simulink model "pod_3_level_V1_2"  (R2018a)
settings: Solver=VariableStepAuto  StartTime=0.0  StopTime=0.1  RelTol=1e-3
libraries: powerlib x24, simulink x6
settings Model: Creator=SuperITCom  LastModifiedBy=SuperITCom

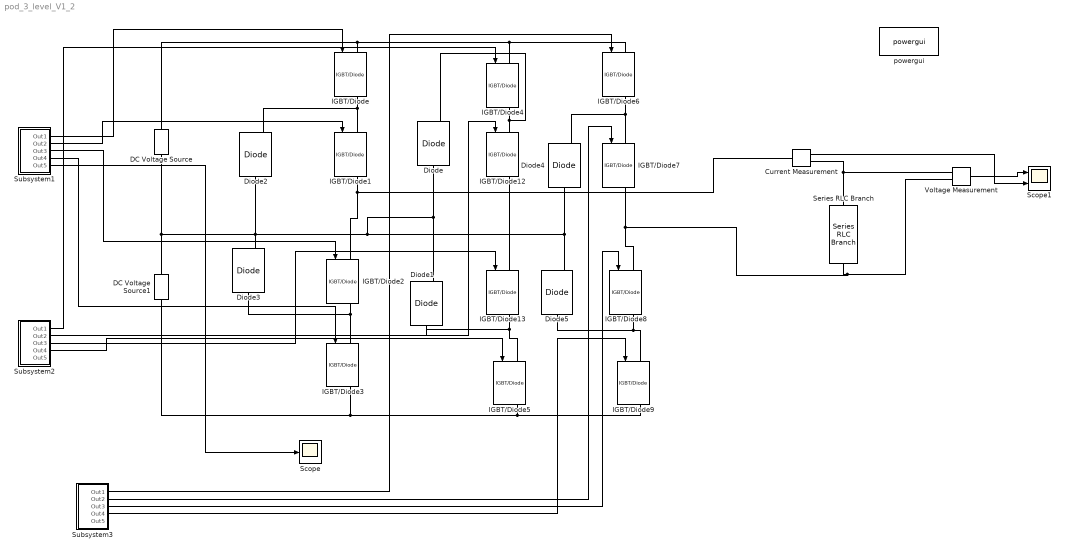
== system pod_3_level_V1_2 ==
  Current Measurement : powerlib/Measurements/Current Measurement  PhasorSimulation=off  OutputType=Complex  PSBequivalent=0
  DC Voltage Source : powerlib/Electrical Sources/DC Voltage Source  Amplitude=200  Measurements=None
  DC Voltage Source1 : powerlib/Electrical Sources/DC Voltage Source  Amplitude=200  Measurements=None
  Diode{,1..5} (6 alike) : powerlib/Power Electronics/Diode  Ron=0.001  Lon=0  Vf=0.8  IC=0  UseSnubber=0  Rs=500  Cs=250e-9  Measurements=on
  IGBT/Diode{,1..9,12..13} (12 alike) : powerlib/Power Electronics/IGBT//Diode  Ron=1e-3  Rs=1e5  Cs=inf  Measurements=on
  Scope : Scope
  Scope1 : Scope  NumInputPorts=2
  Series RLC Branch : powerlib/Elements/Series RLC Branch  LConnTagsString=__new0  RConnTagsString=__new0  BranchType=RL  Resistance=5  Inductance=5e-3  SetiL0=off  InitialCurrent=0  Capacitance=5e-3  Setx0=off  InitialVoltage=0  Measurements=None
  Subsystem1 : Subsystem
  Subsystem2 : Subsystem
  Subsystem3 : Subsystem
  Voltage Measurement : powerlib/Measurements/Voltage Measurement  PhasorSimulation=off  OutputType=Complex  PSBequivalent=0
  powergui : powerlib/powergui  Priority=1  SimulationMode=Discrete  SampleTime=50e-6  frequency=60  Iterations=50  frequencyindice=0  Pbase=100e6  ErrMax=1e-4  UnitsV=kV  UnitsW=MW  buscounter=0  FunctionMessages=off  echomessages=off  EnableUseOfTLC=off  CurrentSourceSwitches=off  DisableSnubberDevices=off  DisableRonSwitches=off  DisableVfSwitches=off  DisplayEquations=off  SolverType=Tustin/Backward Euler (TBE)  Interpol=off  ExternalGateDelay=off  methode=off  Ts=100  x0status=blocks  SPID=off  SwTol=0  HookPort=off  RestoreLinks=warning  ResistiveCurrentMeasurement=off  Frange=[0:2:500]  Ylog=off  Xlog=on  ShowGrid=off  save=off  variable=ZData  structure=linevoltpod3  ZoomFFT=on  StartTime=0.0  cycles=2  DisplayStyle=1  fundamental=50  FreqAxis=on  MaxFrequency=1000  frequencyindicesteady=1  RmsSteady=1  display=off
  wires:
  Current Measurement/1 -> Scope1/2
  Subsystem2/3(Out3) -> IGBT/Diode13/1
  Subsystem1/2(Out2) -> IGBT/Diode1/1
  Subsystem1/5(Out5) -> Scope/1
  Subsystem3/3(Out3) -> IGBT/Diode8/1
  Subsystem1/4(Out4) -> IGBT/Diode3/1
  Subsystem2/4(Out4) -> IGBT/Diode5/1
  Voltage Measurement/1 -> Scope1/1
  Subsystem1/1(Out1) -> IGBT/Diode/1
  Subsystem2/2(Out2) -> IGBT/Diode12/1
  Subsystem3/1(Out1) -> IGBT/Diode6/1
  Subsystem3/4(Out4) -> IGBT/Diode9/1
  Subsystem1/3(Out3) -> IGBT/Diode2/1
  Subsystem3/2(Out2) -> IGBT/Diode7/1
  Subsystem2/1(Out1) -> IGBT/Diode4/1
  connections:
  IGBT/Diode/LConn1 -- DC Voltage Source/RConn1 -- IGBT/Diode4/LConn1 -- IGBT/Diode6/LConn1
  Diode2/LConn1 -- Diode1/RConn1 -- Diode/LConn1 -- Diode4/LConn1 -- Diode5/RConn1 -- DC Voltage Source1/RConn1 -- DC Voltage Source/LConn1 -- Diode3/RConn1
  IGBT/Diode5/RConn1 -- IGBT/Diode3/RConn1 -- DC Voltage Source1/LConn1 -- IGBT/Diode9/RConn1
  IGBT/Diode12/LConn1 -- IGBT/Diode4/RConn1 -- Diode/RConn1
  IGBT/Diode2/LConn1 -- Current Measurement/LConn1 -- IGBT/Diode1/RConn1
  Series RLC Branch/LConn1 -- Current Measurement/RConn1 -- Voltage Measurement/LConn1
  IGBT/Diode2/RConn1 -- Diode3/LConn1 -- IGBT/Diode3/LConn1
  IGBT/Diode1/LConn1 -- IGBT/Diode/RConn1 -- Diode2/RConn1
  IGBT/Diode5/LConn1 -- IGBT/Diode13/RConn1 -- Diode1/LConn1
  Diode5/LConn1 -- IGBT/Diode9/LConn1 -- IGBT/Diode8/RConn1
  IGBT/Diode7/LConn1 -- IGBT/Diode6/RConn1 -- Diode4/RConn1
  IGBT/Diode12/RConn1 -- IGBT/Diode13/LConn1
  IGBT/Diode7/RConn1 -- Series RLC Branch/RConn1 -- Voltage Measurement/LConn2 -- IGBT/Diode8/LConn1

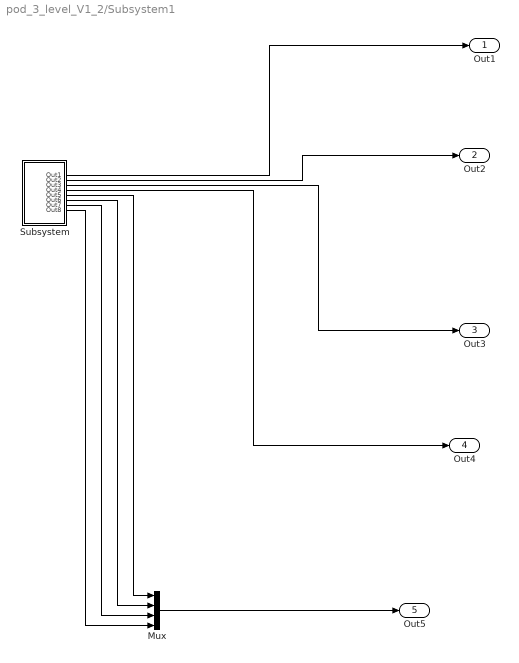
== system pod_3_level_V1_2/Subsystem1 ==
  Mux : Mux
  Subsystem : Subsystem
  Out1 : Outport
  Out2 : Outport  Port=2
  Out3 : Outport  Port=3
  Out4 : Outport  Port=4
  Out5 : Outport  Port=5
  wires:
  Subsystem/6(Out6) -> Mux/2
  Subsystem/5(Out5) -> Mux/1
  Subsystem/8(Out8) -> Mux/4
  Subsystem/7(Out7) -> Mux/3
  Subsystem/1(Out1) -> Out1/1
  Mux/1 -> Out5/1
  Subsystem/2(Out2) -> Out2/1
  Subsystem/4(Out4) -> Out4/1
  Subsystem/3(Out3) -> Out3/1

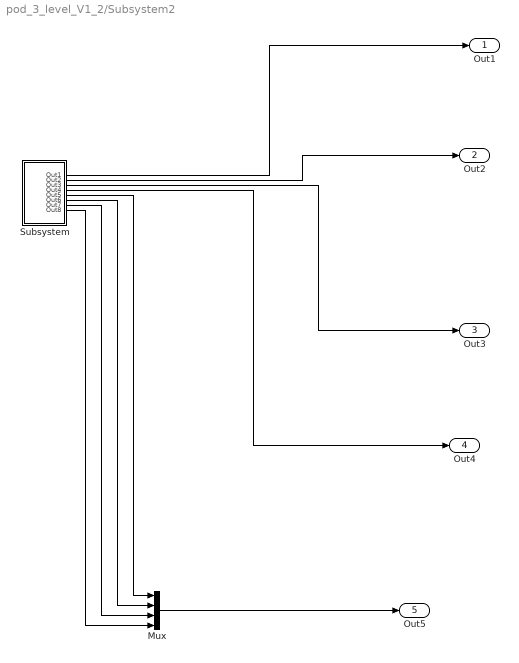
== system pod_3_level_V1_2/Subsystem2 ==
  Mux : Mux
  Subsystem : Subsystem
  Out1 : Outport
  Out2 : Outport  Port=2
  Out3 : Outport  Port=3
  Out4 : Outport  Port=4
  Out5 : Outport  Port=5
  wires:
  Subsystem/6(Out6) -> Mux/2
  Subsystem/5(Out5) -> Mux/1
  Subsystem/8(Out8) -> Mux/4
  Subsystem/7(Out7) -> Mux/3
  Subsystem/1(Out1) -> Out1/1
  Mux/1 -> Out5/1
  Subsystem/2(Out2) -> Out2/1
  Subsystem/4(Out4) -> Out4/1
  Subsystem/3(Out3) -> Out3/1

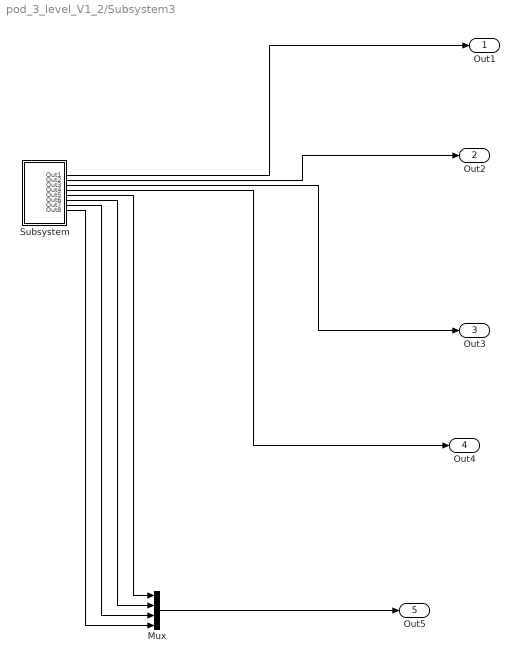
== system pod_3_level_V1_2/Subsystem3 ==
  Mux : Mux
  Subsystem : Subsystem
  Out1 : Outport
  Out2 : Outport  Port=2
  Out3 : Outport  Port=3
  Out4 : Outport  Port=4
  Out5 : Outport  Port=5
  wires:
  Subsystem/6(Out6) -> Mux/2
  Subsystem/5(Out5) -> Mux/1
  Subsystem/8(Out8) -> Mux/4
  Subsystem/7(Out7) -> Mux/3
  Subsystem/1(Out1) -> Out1/1
  Mux/1 -> Out5/1
  Subsystem/2(Out2) -> Out2/1
  Subsystem/4(Out4) -> Out4/1
  Subsystem/3(Out3) -> Out3/1

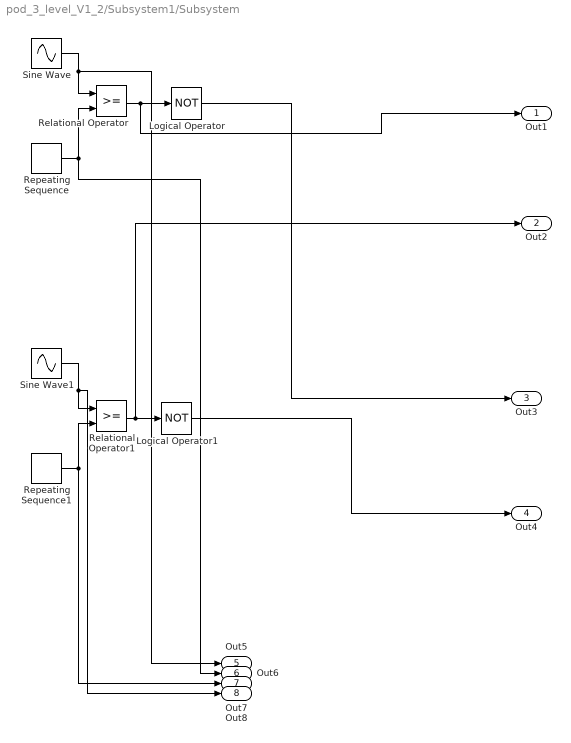
== system pod_3_level_V1_2/Subsystem1/Subsystem ==
  Logical Operator : Logic  Operator=NOT  AllPortsSameDT=off  OutDataTypeStr=boolean
  Logical Operator1 : Logic  Operator=NOT  AllPortsSameDT=off  OutDataTypeStr=boolean
  Relational Operator : RelationalOperator  OutDataTypeStr=boolean  RndMeth=Simplest
  Relational Operator1 : RelationalOperator  OutDataTypeStr=boolean  RndMeth=Simplest
  Repeating Sequence : simulink/Sources/Repeating Sequence  rep_seq_t=[0 0.5 1]/1000  rep_seq_y=[0 1 0]
  Repeating Sequence1 : simulink/Sources/Repeating Sequence  rep_seq_t=[0 0.5 1]/1000  rep_seq_y=[0 -1 0]
  Sine Wave : Sin  Amplitude=1.0  Frequency=2*pi*50  SampleTime=0
  Sine Wave1 : Sin  Amplitude=1.0  Frequency=2*pi*50  SampleTime=0
  Out1 : Outport
  Out2 : Outport  Port=2
  Out3 : Outport  Port=3
  Out4 : Outport  Port=4
  Out5 : Outport  Port=5
  Out6 : Outport  Port=6
  Out7 : Outport  Port=7
  Out8 : Outport  Port=8
  wires:
  Relational Operator1/1 -> Out2/1, Logical Operator1/1
  Repeating Sequence1/1 -> Out7/1, Relational Operator1/2
  Sine Wave1/1 -> Out8/1, Relational Operator1/1
  Relational Operator/1 -> Out1/1, Logical Operator/1
  Repeating Sequence/1 -> Out6/1, Relational Operator/2
  Sine Wave/1 -> Out5/1, Relational Operator/1
  Logical Operator/1 -> Out3/1
  Logical Operator1/1 -> Out4/1

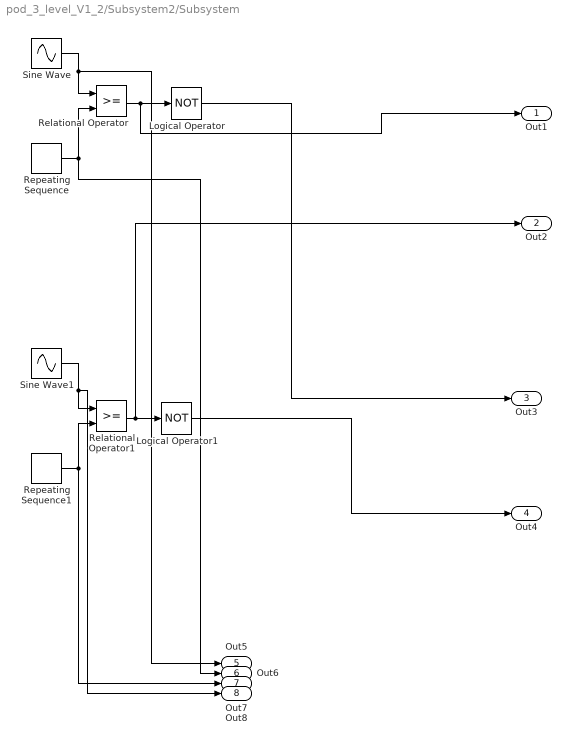
== system pod_3_level_V1_2/Subsystem2/Subsystem ==
  Logical Operator : Logic  Operator=NOT  AllPortsSameDT=off  OutDataTypeStr=boolean
  Logical Operator1 : Logic  Operator=NOT  AllPortsSameDT=off  OutDataTypeStr=boolean
  Relational Operator : RelationalOperator  OutDataTypeStr=boolean  RndMeth=Simplest
  Relational Operator1 : RelationalOperator  OutDataTypeStr=boolean  RndMeth=Simplest
  Repeating Sequence : simulink/Sources/Repeating Sequence  rep_seq_t=[0 0.5 1]/1000  rep_seq_y=[0 1 0]
  Repeating Sequence1 : simulink/Sources/Repeating Sequence  rep_seq_t=[0 0.5 1]/1000  rep_seq_y=[0 -1 0]
  Sine Wave : Sin  Amplitude=1.0  Frequency=2*pi*50  Phase=(2*pi)/3  SampleTime=0
  Sine Wave1 : Sin  Amplitude=1.0  Frequency=2*pi*50  Phase=(2*pi)/3  SampleTime=0
  Out1 : Outport
  Out2 : Outport  Port=2
  Out3 : Outport  Port=3
  Out4 : Outport  Port=4
  Out5 : Outport  Port=5
  Out6 : Outport  Port=6
  Out7 : Outport  Port=7
  Out8 : Outport  Port=8
  wires:
  Relational Operator1/1 -> Out2/1, Logical Operator1/1
  Repeating Sequence1/1 -> Out7/1, Relational Operator1/2
  Sine Wave1/1 -> Out8/1, Relational Operator1/1
  Relational Operator/1 -> Out1/1, Logical Operator/1
  Repeating Sequence/1 -> Out6/1, Relational Operator/2
  Sine Wave/1 -> Out5/1, Relational Operator/1
  Logical Operator/1 -> Out3/1
  Logical Operator1/1 -> Out4/1

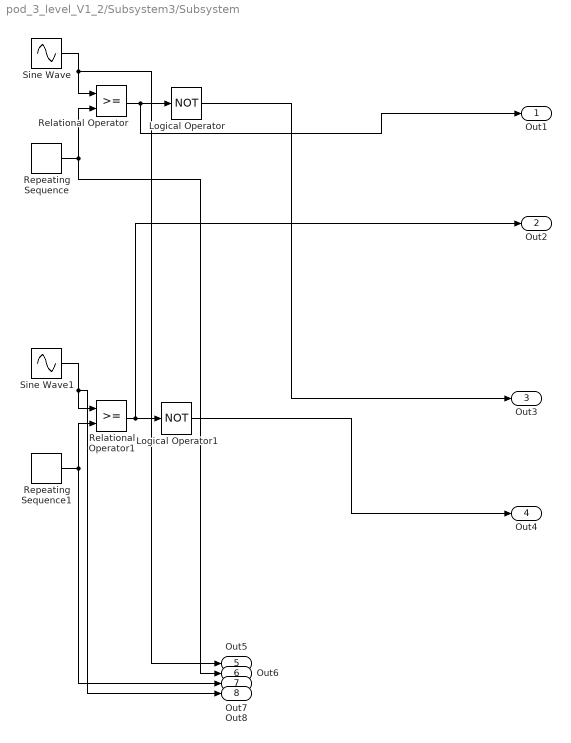
== system pod_3_level_V1_2/Subsystem3/Subsystem ==
  Logical Operator : Logic  Operator=NOT  AllPortsSameDT=off  OutDataTypeStr=boolean
  Logical Operator1 : Logic  Operator=NOT  AllPortsSameDT=off  OutDataTypeStr=boolean
  Relational Operator : RelationalOperator  OutDataTypeStr=boolean  RndMeth=Simplest
  Relational Operator1 : RelationalOperator  OutDataTypeStr=boolean  RndMeth=Simplest
  Repeating Sequence : simulink/Sources/Repeating Sequence  rep_seq_t=[0 0.5 1]/1000  rep_seq_y=[0 1 0]
  Repeating Sequence1 : simulink/Sources/Repeating Sequence  rep_seq_t=[0 0.5 1]/1000  rep_seq_y=[0 -1 0]
  Sine Wave : Sin  Amplitude=1.0  Frequency=2*pi*50  Phase=(4*pi)/3  SampleTime=0
  Sine Wave1 : Sin  Amplitude=1.0  Frequency=2*pi*50  Phase=(4*pi)/3  SampleTime=0
  Out1 : Outport
  Out2 : Outport  Port=2
  Out3 : Outport  Port=3
  Out4 : Outport  Port=4
  Out5 : Outport  Port=5
  Out6 : Outport  Port=6
  Out7 : Outport  Port=7
  Out8 : Outport  Port=8
  wires:
  Relational Operator1/1 -> Out2/1, Logical Operator1/1
  Repeating Sequence1/1 -> Out7/1, Relational Operator1/2
  Sine Wave1/1 -> Out8/1, Relational Operator1/1
  Relational Operator/1 -> Out1/1, Logical Operator/1
  Repeating Sequence/1 -> Out6/1, Relational Operator/2
  Sine Wave/1 -> Out5/1, Relational Operator/1
  Logical Operator/1 -> Out3/1
  Logical Operator1/1 -> Out4/1
